simulink model "Motore_corrente_continua_simulink"  (R2022b)
settings: Solver=VariableStepAuto  StartTime=0.0  StopTime=10.0  RelTol=1e-3
values from neighbouring files (symbols this model uses):
  b = 1    [Motore_corrente_continua.m]    (also in Motore_workspace.m = 100)
  j = 1    [Motore_corrente_continua.m]    (also in Motore_workspace.m = 200)
  Kv = 1    [Motore_corrente_continua.m]    (also in Motore_workspace.m = 0.1)
  l = 1    [Motore_corrente_continua.m]    (also in Motore_workspace.m = 100)
  r = 1    [Motore_corrente_continua.m]    (also in Motore_workspace.m = 100)
  v = 10    [Motore_corrente_continua.m]    (also in Motore_workspace.m = 2)
settings Model: Creator=giuli  LastModifiedBy=giuli

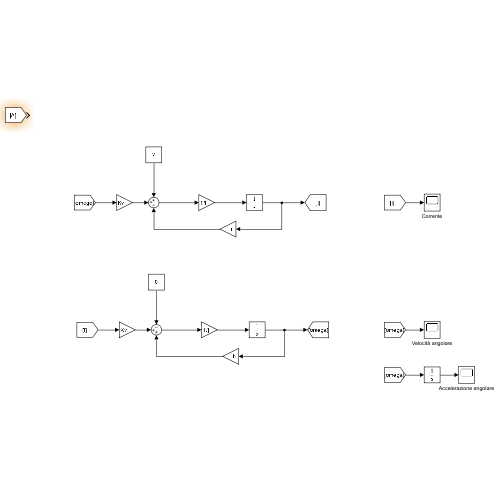
[thumbnail: Simulink's stored preview of the top-level diagram]
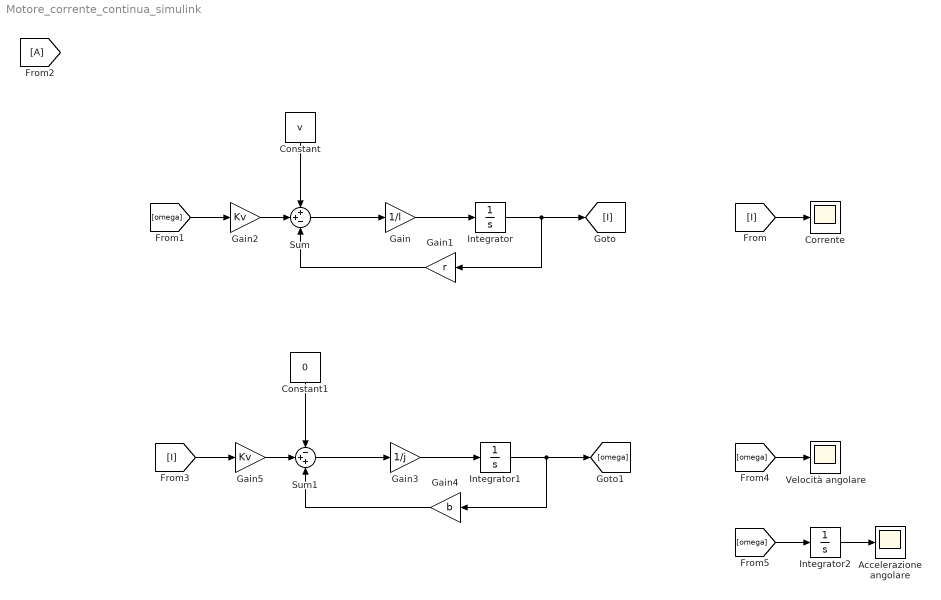
== system Motore_corrente_continua_simulink ==
  Accelerazione angolare : Scope
  Constant : Constant  Value=v
  Constant1 : Constant  Value=0
  Corrente : Scope
  From2 : From
  Gain : Gain  Gain=1/l
  Gain1 : Gain  Gain=r
  Gain2 : Gain  Gain=Kv
  Gain3 : Gain  Gain=1/j
  Gain4 : Gain  Gain=b
  Gain5 : Gain  Gain=Kv
  Integrator : Integrator
  Integrator1 : Integrator
  Integrator2 : Integrator
  Sum : Sum  Inputs=++-
  Sum1 : Sum  Inputs=-++
  Velocità angolare : Scope
  wires:
  Integrator/1 -> Gain1/1, [I]
  Gain/1 -> Integrator/1
  Sum/1 -> Gain/1
  Gain1/1 -> Sum/3
  Constant/1 -> Sum/1
  Gain2/1 -> Sum/2
  [omega] -> Gain2/1
  [I] -> Gain5/1
  Gain3/1 -> Integrator1/1
  Constant1/1 -> Sum1/1
  Gain4/1 -> Sum1/3
  Gain5/1 -> Sum1/2
  Integrator1/1 -> Gain4/1, [omega]
  Sum1/1 -> Gain3/1
  [I] -> Corrente/1
  [omega] -> Velocità angolare/1
  Integrator2/1 -> Accelerazione angolare/1
  [omega] -> Integrator2/1
